simulink model "ROS_LQT"  (R2015b)
settings: Solver=VariableStepAuto  StartTime=0.0  StopTime=tsim+1  RelTol=1e-3
values from neighbouring files (symbols this model uses):
  A_kal = [1 0 0 Ts 0 0 ... (first row only)    [LQT_12states.m]
  C_kal = [1 0 0 0 0 0 ... (first row only)    [LQT_12states.m]
  Ki_LQT = [Ki_coef  -Ki_coef   -Ki_coefz ... (first row only)    [LQT_12states.m]
  R_kal = diag([5e-9 5e-9 5e-9])    [LQT_12states.m]
  Ts = 0.01    [LQT_12states.m]    (also in Trajectory_generation.m)
  tsim = 40    [LQT_12states.m]
undefined symbols (not defined in the file or in its folder): Angular, DiscIntNeverNeededParam, Discrete, Linear, pwm, Time
libraries: simulink x6, robotlib x5, realtime_pacer_lib x2, ctrlSharedLib x1, aerolibtransform2 x1
settings Model: Creator=carlosluis  LastModifiedBy=carlosluis

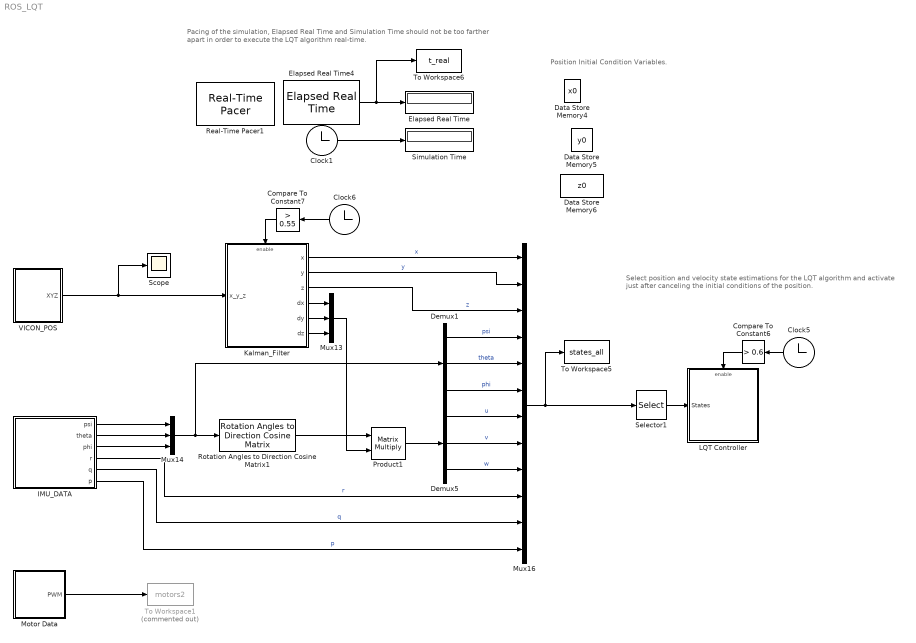
== system ROS_LQT ==
  note: Select position and velocity state estimations for the LQT
      | algorithm and activate just after canceling the initial
      | conditions of the position.
  note: Pacing of the simulation, Elapsed Real Time and Simulation Time should
      | not be too farther apart in order to execute the LQT algorithm real-time.
  note: Position Initial Condition Variables.
  Clock1 : Clock
  Clock5 : Clock
  Clock6 : Clock
  Compare To Constant6 : simulink/Logic and Bit Operations/Compare To Constant  relop=>  const=0.6  OutDataTypeStr=boolean
  Compare To Constant7 : simulink/Logic and Bit Operations/Compare To Constant  relop=>  const=0.55  OutDataTypeStr=boolean
  Data Store Memory4 : DataStoreMemory  DataStoreName=x0  ReadBeforeWriteMsg=warning  WriteAfterWriteMsg=warning  WriteAfterReadMsg=warning  OutDataTypeStr=double
  Data Store Memory5 : DataStoreMemory  DataStoreName=y0  ReadBeforeWriteMsg=warning  WriteAfterWriteMsg=warning  WriteAfterReadMsg=warning  OutDataTypeStr=double
  Data Store Memory6 : DataStoreMemory  DataStoreName=z0  ReadBeforeWriteMsg=warning  WriteAfterWriteMsg=warning  WriteAfterReadMsg=warning  OutDataTypeStr=double
  Demux1 : Demux  Outputs=3
  Demux5 : Demux  Outputs=3
  Elapsed Real Time : Display
      settings: Decimation=2
  Elapsed Real Time4 : realtime_pacer_lib/Elapsed Real Time
  IMU_DATA : Subsystem
  Kalman_Filter : Subsystem
  LQT Controller : Subsystem
  Motor Data : Subsystem
  Mux13 : Mux  Inputs=3
  Mux14 : Mux  Inputs=3
  Mux16 : Mux  Inputs=12
  Product1 : Product  Multiplication=Matrix(*)
  Real-Time Pacer1 : realtime_pacer_lib/Real-Time Pacer  simTimePerRealTime=1
  Rotation Angles to Direction Cosine Matrix1 : aerolibtransform2/Rotation Angles to Direction Cosine Matrix  rotationOrder=ZYX
  Scope : Scope
  Selector1 : Selector  InputPortWidth=12  IndexOptions=Index vector (dialog)  Indices=[1 2 3 7 8 9]  OutputSizes=1
  Simulation Time : Display
      settings: Decimation=2
  To Workspace1 : ToWorkspace  Commented=on  VariableName=motors2  SampleTime=Ts
  To Workspace5 : ToWorkspace  VariableName=states_all  SampleTime=Ts
  To Workspace6 : ToWorkspace  VariableName=t_real  SampleTime=Ts
  VICON_POS : Subsystem
  wires:
  Elapsed Real Time4/1 -> Elapsed Real Time/1, To Workspace6/1
  Mux14/1 -> Demux1/1, Rotation Angles to Direction Cosine Matrix1/1
  Rotation Angles to Direction Cosine Matrix1/1 -> Product1/1
  Product1/1 -> Demux5/1
  Compare To Constant6/1 -> LQT Controller/Enable
  Clock6/1 -> Compare To Constant7/1
  Compare To Constant7/1 -> Kalman_Filter/Enable
  Clock5/1 -> Compare To Constant6/1
  Selector1/1 -> LQT Controller/1(States)
  Kalman_Filter/4(dx) -> Mux13/1
  Kalman_Filter/5(dy) -> Mux13/2
  Kalman_Filter/6(dz) -> Mux13/3
  IMU_DATA/1(psi) -> Mux14/1
  IMU_DATA/2(theta) -> Mux14/2
  IMU_DATA/3(phi) -> Mux14/3
  Mux13/1 -> Product1/2
  Kalman_Filter/1(x) -> Mux16/1  "x"
  Kalman_Filter/2(y) -> Mux16/2  "y"
  Kalman_Filter/3(z) -> Mux16/3  "z"
  IMU_DATA/4(r) -> Mux16/10  "r"
  IMU_DATA/5(q) -> Mux16/11  "q"
  IMU_DATA/6(p) -> Mux16/12  "p"
  Mux16/1 -> To Workspace5/1, Selector1/1
  Demux5/1 -> Mux16/7  "u"
  Demux5/2 -> Mux16/8  "v"
  Demux5/3 -> Mux16/9  "w"
  Demux1/1 -> Mux16/4  "psi"
  Demux1/2 -> Mux16/5  "theta"
  Demux1/3 -> Mux16/6  "phi"
  Motor Data/1(PWM) -> To Workspace1/1
  Clock1/1 -> Simulation Time/1
  VICON_POS/1(XYZ) -> Scope/1, Kalman_Filter/1(x_y_z)

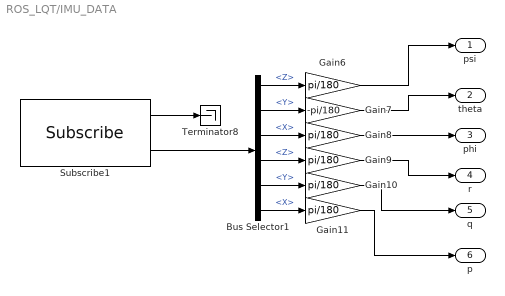
== system ROS_LQT/IMU_DATA ==
  Bus Selector1 : BusSelector  OutputSignals=AngularVelocity.Z,AngularVelocity.Y,AngularVelocity.X,LinearAcceleration.Z,LinearAcceleration.Y,LinearAcceleration.X
  Gain{6,8..11} (5 alike) : Gain  Gain=pi/180
  Gain7 : Gain  Gain=-pi/180
  Subscribe1 : robotlib/Subscribe  SourceLibraryInfo=This block requires Robotics System Toolbox  topicSource=Specify your own  topic=/crazyflie/imu  messageType=sensor_msgs/Imu  sampleTime=1/50  messageQueueLength=1
  Terminator8 : Terminator
  psi : Outport
  theta : Outport  Port=2
  phi : Outport  Port=3
  r : Outport  Port=4
  q : Outport  Port=5
  p : Outport  Port=6
  wires:
  Gain11/1 -> p/1
  Gain10/1 -> q/1
  Gain9/1 -> r/1
  Subscribe1/2 -> Bus Selector1/1
  Subscribe1/1 -> Terminator8/1
  Bus Selector1/3 -> Gain8/1  "<X>"
  Bus Selector1/2 -> Gain7/1  "<Y>"
  Bus Selector1/1 -> Gain6/1  "<Z>"
  Bus Selector1/4 -> Gain9/1  "<Z>"
  Bus Selector1/5 -> Gain10/1  "<Y>"
  Bus Selector1/6 -> Gain11/1  "<X>"
  Gain7/1 -> theta/1
  Gain8/1 -> phi/1
  Gain6/1 -> psi/1

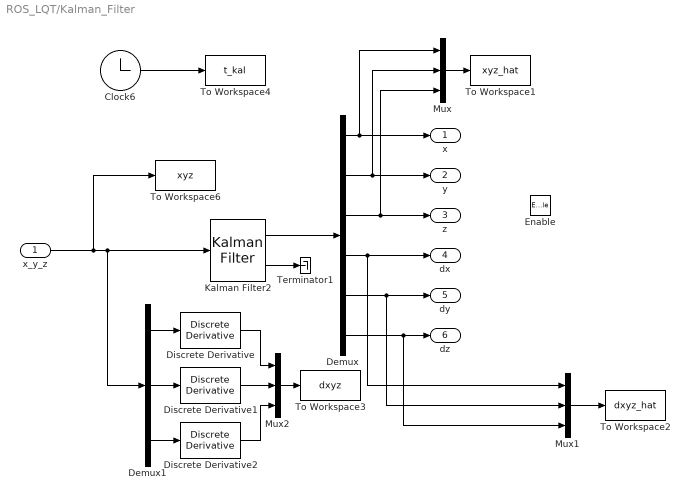
== system ROS_LQT/Kalman_Filter ==
  x_y_z : Inport
  Enable : EnablePort
  Clock6 : Clock
  Demux : Demux  Outputs=6
  Demux1 : Demux  Outputs=3
  Discrete Derivative : simulink/Discrete/Discrete Derivative  gainval=1.0  ICPrevScaledInput=0.0  InputProcessing=Inherited  OutMin=[]  OutMax=[]  OutDataType=fixdt(1, 16)  OutScaling=2^-10  DoSatur=off
  Discrete Derivative1 : simulink/Discrete/Discrete Derivative  gainval=1.0  ICPrevScaledInput=0.0  InputProcessing=Inherited  OutMin=[]  OutMax=[]  OutDataType=fixdt(1, 16)  OutScaling=2^-10  DoSatur=off
  Discrete Derivative2 : simulink/Discrete/Discrete Derivative  gainval=1.0  ICPrevScaledInput=0.0  InputProcessing=Inherited  OutMin=[]  OutMax=[]  OutDataType=fixdt(1, 16)  OutScaling=2^-10  DoSatur=off
  Kalman Filter2 : ctrlSharedLib/Kalman Filter  TimeDomain=Discrete-Time  UseCurrentEstimator=on  ModelSource=Individual A, B, C, D matrices  ModelSourceVariable=ss(0.95,1,1,0,1)  A=A_kal  B=1  C=C_kal  D=0  NumberOfStates=1  NumberOfInputs=1  NumberOfOutputs=1  InitialEstimateSource=Dialog  X0=0  P0=10  UseK=off  UseGH=on  NumberOfProcessNoiseInputs=1  G=G_kal  TimeInvariantG=on  H=0  TimeInvariantH=on  Q=Q_kal  TimeInvariantQ=on  R=R_kal  TimeInvariantR=on  N=0  TimeInvariantN=on  AddInputPort=off  AddEnablePort=off  OutputEstimatedY=off  OutputP=on  Ts=Ts
  Mux : Mux  Inputs=3
  Mux1 : Mux  Inputs=3
  Mux2 : Mux  Inputs=3
  Terminator1 : Terminator
  To Workspace1 : ToWorkspace  VariableName=xyz_hat  SampleTime=Ts
  To Workspace2 : ToWorkspace  VariableName=dxyz_hat  SampleTime=Ts
  To Workspace3 : ToWorkspace  VariableName=dxyz  SampleTime=Ts
  To Workspace4 : ToWorkspace  VariableName=t_kal  SampleTime=Ts
  To Workspace6 : ToWorkspace  VariableName=xyz  SampleTime=Ts
  x : Outport
  y : Outport  Port=2
  z : Outport  Port=3
  dx : Outport  Port=4
  dy : Outport  Port=5
  dz : Outport  Port=6
  wires:
  Demux/6 -> Mux1/3, dz/1
  Demux/5 -> Mux1/2, dy/1
  Demux/4 -> Mux1/1, dx/1
  Demux/2 -> Mux/2, y/1
  Demux/3 -> Mux/3, z/1
  Kalman Filter2/1 -> Demux/1
  Demux/1 -> Mux/1, x/1
  x_y_z/1 -> To Workspace6/1, Demux1/1, Kalman Filter2/1
  Kalman Filter2/2 -> Terminator1/1
  Mux/1 -> To Workspace1/1
  Mux1/1 -> To Workspace2/1
  Mux2/1 -> To Workspace3/1
  Clock6/1 -> To Workspace4/1
  Demux1/3 -> Discrete Derivative2/1
  Discrete Derivative2/1 -> Mux2/3
  Demux1/2 -> Discrete Derivative1/1
  Discrete Derivative1/1 -> Mux2/2
  Discrete Derivative/1 -> Mux2/1
  Demux1/1 -> Discrete Derivative/1

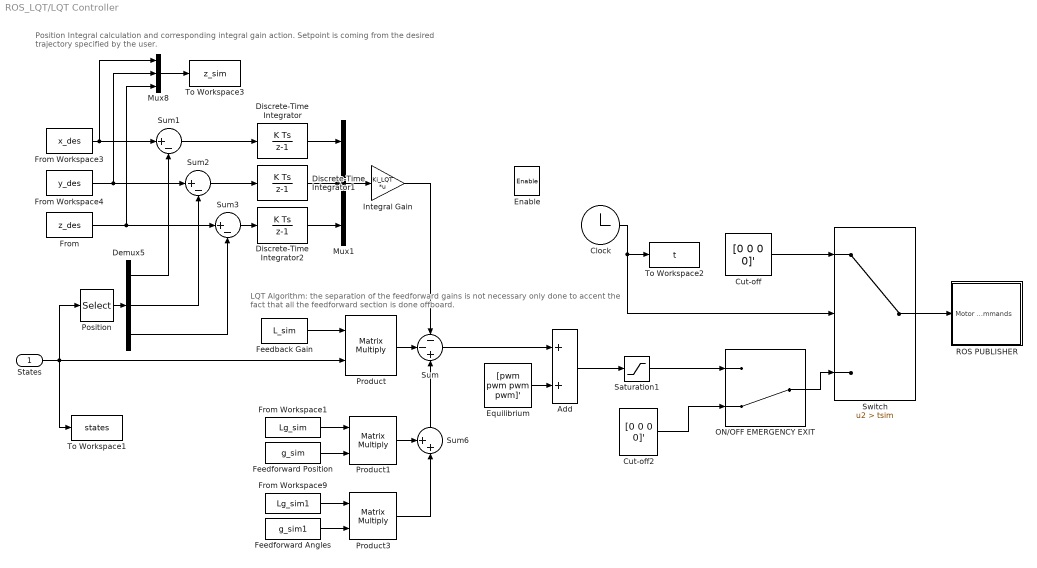
== system ROS_LQT/LQT Controller ==
  note: LQT Algorithm: the separation of the feedforward gains is not necessary
      | only done to accent the fact that all the feedforward section is done offboard.
  note: Position Integral calculation and corresponding integral gain action. Setpoint is coming
      | from the desired trajectory specified by the user.
  States : Inport
  Enable : EnablePort
  Add : Sum
  Clock : Clock
  Cut-off : Constant  Value=[0 0 0 0]'
  Cut-off2 : Constant  Value=[0 0 0 0]'
  Demux5 : Demux  Outputs=3
  Discrete-Time Integrator : DiscreteIntegrator  gainval=1  InitialConditionSetting=State (most efficient)  SampleTime=Ts  LimitOutput=on  UpperSaturationLimit=1000  LowerSaturationLimit=-1000  ICPrevOutput=DiscIntNeverNeededParam  ICPrevScaledInput=DiscIntNeverNeededParam
  Discrete-Time Integrator1 : DiscreteIntegrator  gainval=1  InitialConditionSetting=State (most efficient)  SampleTime=Ts  LimitOutput=on  UpperSaturationLimit=1000  LowerSaturationLimit=-1000  ICPrevOutput=DiscIntNeverNeededParam  ICPrevScaledInput=DiscIntNeverNeededParam
  Discrete-Time Integrator2 : DiscreteIntegrator  gainval=1  InitialConditionSetting=State (most efficient)  SampleTime=Ts  LimitOutput=on  UpperSaturationLimit=1000  LowerSaturationLimit=-1000  ICPrevOutput=DiscIntNeverNeededParam  ICPrevScaledInput=DiscIntNeverNeededParam
  Equilibrium : Constant  Value=[pwm pwm pwm pwm]'
  Feedback Gain : FromWorkspace  VariableName=L_sim  SampleTime=Ts
  Feedforward Angles : FromWorkspace  VariableName=g_sim1  SampleTime=Ts
  "Feedforward Position " : FromWorkspace  VariableName=g_sim  SampleTime=Ts
  From : FromWorkspace  VariableName=z_des  SampleTime=Ts
  From Workspace1 : FromWorkspace  VariableName=Lg_sim  SampleTime=Ts
  From Workspace3 : FromWorkspace  VariableName=x_des  SampleTime=Ts
  From Workspace4 : FromWorkspace  VariableName=y_des  SampleTime=Ts
  From Workspace9 : FromWorkspace  VariableName=Lg_sim1  SampleTime=Ts
  Integral Gain : Gain  Gain=Ki_LQT  Multiplication=Matrix(K*u)
  Mux1 : Mux  Inputs=3
  Mux8 : Mux  Inputs=3
  ON/OFF EMERGENCY EXIT : ManualSwitch  CurrentSetting=0
  Position : Selector  InputPortWidth=6  IndexOptions=Index vector (dialog)  Indices=[1 2 3]  OutputSizes=1
  Product : Product  Multiplication=Matrix(*)
  Product1 : Product  Multiplication=Matrix(*)
  Product3 : Product  Multiplication=Matrix(*)
  ROS PUBLISHER : Subsystem
  Saturation1 : Saturate  UpperLimit=60000
  Sum : Sum  Inputs=--+
  Sum1 : Sum  Inputs=|+-
  Sum2 : Sum  Inputs=|+-
  Sum3 : Sum  Inputs=|+-
  Sum6 : Sum  Inputs=++|
  Switch : Switch  Criteria=u2 > Threshold  Threshold=tsim
  To Workspace1 : ToWorkspace  VariableName=states  SampleTime=Ts
  To Workspace2 : ToWorkspace  VariableName=t  SampleTime=Ts
  To Workspace3 : ToWorkspace  VariableName=z_sim  SampleTime=Ts
  wires:
  Cut-off/1 -> Switch/1
  From Workspace1/1 -> Product1/1
  "Feedforward Position "/1 -> Product1/2
  Feedback Gain/1 -> Product/1
  Add/1 -> Saturation1/1
  From Workspace3/1 -> Mux8/1, Sum1/1
  From Workspace4/1 -> Mux8/2, Sum2/1
  Sum1/1 -> Discrete-Time Integrator/1
  Sum2/1 -> Discrete-Time Integrator1/1
  Mux8/1 -> To Workspace3/1
  Equilibrium/1 -> Add/2
  From/1 -> Mux8/3, Sum3/1
  Sum3/1 -> Discrete-Time Integrator2/1
  From Workspace9/1 -> Product3/1
  Feedforward Angles/1 -> Product3/2
  Sum/1 -> Add/1
  Discrete-Time Integrator/1 -> Mux1/1
  Discrete-Time Integrator1/1 -> Mux1/2
  Discrete-Time Integrator2/1 -> Mux1/3
  Mux1/1 -> Integral Gain/1
  States/1 -> Position/1, Product/2, To Workspace1/1
  Position/1 -> Demux5/1
  Demux5/1 -> Sum1/2
  Demux5/2 -> Sum2/2
  Demux5/3 -> Sum3/2
  Product1/1 -> Sum6/1
  Product3/1 -> Sum6/2
  Product/1 -> Sum/2
  Integral Gain/1 -> Sum/1
  Sum6/1 -> Sum/3
  Clock/1 -> Switch/2, To Workspace2/1
  Saturation1/1 -> ON/OFF EMERGENCY EXIT/1
  Cut-off2/1 -> ON/OFF EMERGENCY EXIT/2
  ON/OFF EMERGENCY EXIT/1 -> Switch/3
  Switch/1 -> ROS PUBLISHER/1(Motor Commands)

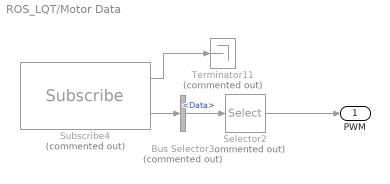
== system ROS_LQT/Motor Data ==
  Bus Selector3 : BusSelector  Commented=on  OutputSignals=Data
  Selector2 : Selector  Commented=on  InputPortWidth=128  IndexOptions=Index vector (dialog)  Indices=[1 2 3 4]  OutputSizes=1
  Subscribe4 : robotlib/Subscribe  Commented=on  SourceLibraryInfo=This block requires Robotics System Toolbox  topicSource=Specify your own  topic=/crazyflie/motor  messageType=std_msgs/Int32MultiArray  sampleTime=0.1  messageQueueLength=1
  Terminator11 : Terminator  Commented=on
  PWM : Outport
  wires:
  Subscribe4/1 -> Terminator11/1
  Selector2/1 -> PWM/1
  Subscribe4/2 -> Bus Selector3/1
  Bus Selector3/1 -> Selector2/1  "<Data>"

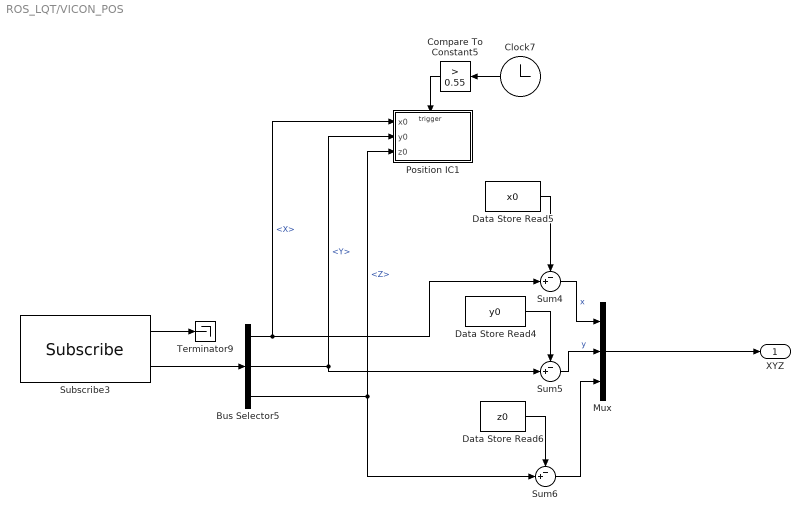
== system ROS_LQT/VICON_POS ==
  Bus Selector5 : BusSelector  OutputSignals=X,Y,Z
  Clock7 : Clock
  Compare To Constant5 : simulink/Logic and Bit Operations/Compare To Constant  relop=>  const=0.55  OutDataTypeStr=boolean
  Data Store Read4 : DataStoreRead  DataStoreName=y0  SampleTime=Ts
  Data Store Read5 : DataStoreRead  DataStoreName=x0  SampleTime=Ts
  Data Store Read6 : DataStoreRead  DataStoreName=z0  SampleTime=Ts
  Mux : Mux  Inputs=3
  Position IC1 : Subsystem
  Subscribe3 : robotlib/Subscribe  SourceLibraryInfo=This block requires Robotics System Toolbox  topicSource=Specify your own  topic=/vicon/pos  messageType=geometry_msgs/Vector3  sampleTime=Ts  messageQueueLength=1
  Sum4 : Sum  Inputs=-+|
  Sum5 : Sum  Inputs=-+|
  Sum6 : Sum  Inputs=-+|
  Terminator9 : Terminator
  XYZ : Outport
  wires:
  Bus Selector5/2 -> Sum5/2, Position IC1/2(y0)  "<Y>"
  Bus Selector5/1 -> Sum4/2, Position IC1/1(x0)  "<X>"
  Bus Selector5/3 -> Sum6/2, Position IC1/3(z0)  "<Z>"
  Subscribe3/2 -> Bus Selector5/1
  Subscribe3/1 -> Terminator9/1
  Compare To Constant5/1 -> Position IC1/Trigger
  Clock7/1 -> Compare To Constant5/1
  Data Store Read5/1 -> Sum4/1
  Data Store Read4/1 -> Sum5/1
  Data Store Read6/1 -> Sum6/1
  Sum4/1 -> Mux/1  "x"
  Sum5/1 -> Mux/2  "y"
  Mux/1 -> XYZ/1
  Sum6/1 -> Mux/3

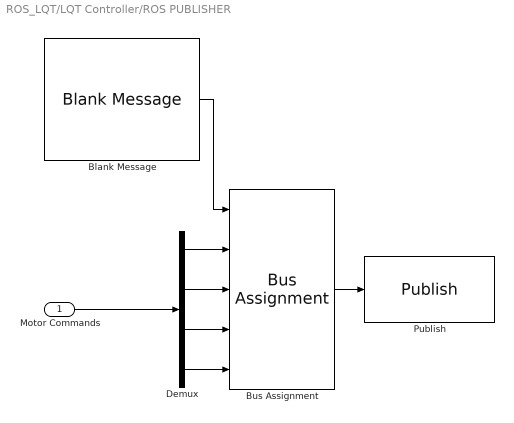
== system ROS_LQT/LQT Controller/ROS PUBLISHER ==
  Motor Commands : Inport
  Blank Message : robotlib/Blank Message  SourceLibraryInfo=This block requires Robotics System Toolbox  messageType=geometry_msgs/Twist  SampleTime=inf
  Bus Assignment : BusAssignment  AssignedSignals=Linear.X,Linear.Y,Linear.Z,Angular.Z
  Demux : Demux
  Publish : robotlib/Publish  SourceLibraryInfo=This block requires Robotics System Toolbox  topicSource=Specify your own  topic=/goal  messageType=geometry_msgs/Twist  messageQueueLength=1
  wires:
  Blank Message/1 -> Bus Assignment/1
  Bus Assignment/1 -> Publish/1
  Motor Commands/1 -> Demux/1
  Demux/1 -> Bus Assignment/2
  Demux/2 -> Bus Assignment/3
  Demux/3 -> Bus Assignment/4
  Demux/4 -> Bus Assignment/5

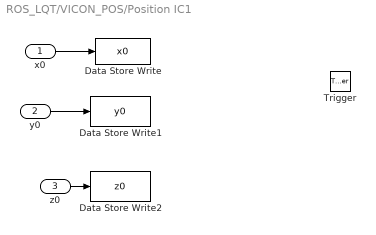
== system ROS_LQT/VICON_POS/Position IC1 ==
  x0 : Inport
  y0 : Inport  Port=2
  z0 : Inport  Port=3
  Trigger : TriggerPort  PortDimensions=1
  Data Store Write : DataStoreWrite  DataStoreName=x0
  Data Store Write1 : DataStoreWrite  DataStoreName=y0
  Data Store Write2 : DataStoreWrite  DataStoreName=z0
  wires:
  x0/1 -> Data Store Write/1
  y0/1 -> Data Store Write1/1
  z0/1 -> Data Store Write2/1
